simulink model "stp5"  (R2016b)
settings: Solver=VariableStepAuto  StartTime=0.0  StopTime=10.0  RelTol=1e-3
undefined symbols (not defined in the file): Ad2, Bd2, Kd, T, X0
settings Model: Creator=arq  LastModifiedBy=arq

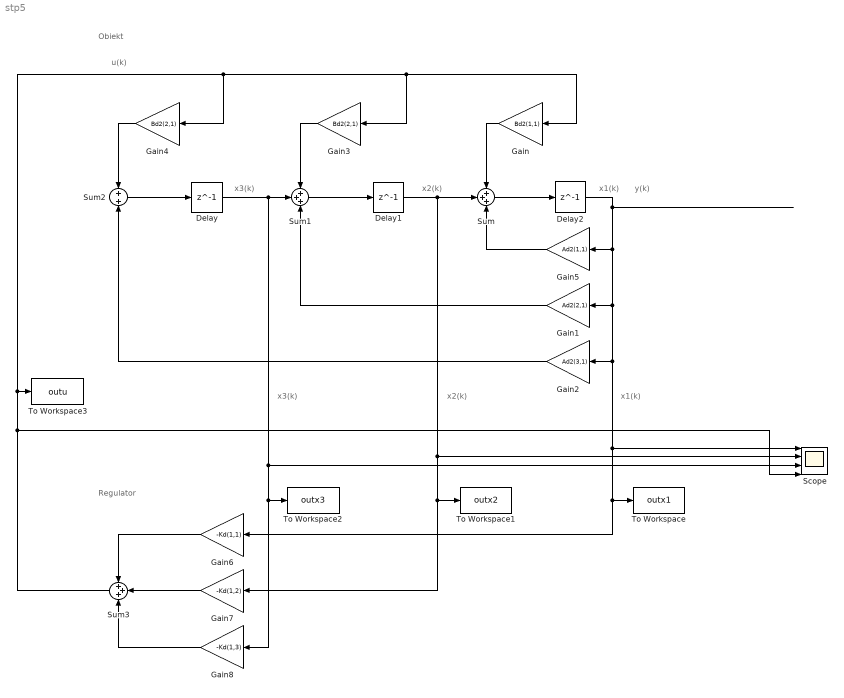
== system stp5 ==
  note: Regulator
  note: Obiekt
  note: u(k)
  note: x3(k)
  note: x2(k)
  note: x1(k)
  note: y(k)
  note: x3(k)
  note: x2(k)
  note: x1(k)
  Delay : Delay  DelayLength=1  InitialCondition=X0(3,1)  SampleTime=T
  Delay1 : Delay  DelayLength=1  InitialCondition=X0(2,1)  SampleTime=T
  Delay2 : Delay  DelayLength=1  InitialCondition=X0(1,1)  SampleTime=T
  Gain : Gain  Gain=Bd2(1,1)
  Gain1 : Gain  Gain=Ad2(2,1)
  Gain2 : Gain  Gain=Ad2(3,1)
  Gain3 : Gain  Gain=Bd2(2,1)
  Gain4 : Gain  Gain=Bd2(2,1)
  Gain5 : Gain  Gain=Ad2(1,1)
  Gain6 : Gain  Gain=-Kd(1,1)
  Gain7 : Gain  Gain=-Kd(1,2)
  Gain8 : Gain  Gain=-Kd(1,3)
  Scope : Scope  NumInputPorts=4
  Sum : Sum  Inputs=3
  Sum1 : Sum  Inputs=3
  Sum2 : Sum  Inputs=2
  Sum3 : Sum  Inputs=+++
  To Workspace : ToWorkspace  VariableName=outx1  SaveFormat=Timeseries  SampleTime=-1
  To Workspace1 : ToWorkspace  VariableName=outx2  SaveFormat=Timeseries  SampleTime=-1
  To Workspace2 : ToWorkspace  VariableName=outx3  SaveFormat=Timeseries  SampleTime=-1
  To Workspace3 : ToWorkspace  VariableName=outu  SaveFormat=Timeseries  SampleTime=-1
  wires:
  Delay2/1 -> Scope/1, Gain6/1, To Workspace/1, Gain2/1, Gain1/1, Gain5/1
  Sum3/1 -> Scope/4, To Workspace3/1, Gain/1, Gain3/1, Gain4/1
  Delay1/1 -> Sum/2, Scope/2, To Workspace1/1, Gain7/1
  Sum/1 -> Delay2/1
  Sum1/1 -> Delay1/1
  Delay/1 -> Scope/3, To Workspace2/1, Gain8/1, Sum1/2
  Gain5/1 -> Sum/3
  Gain1/1 -> Sum1/3
  Gain2/1 -> Sum2/2
  Sum2/1 -> Delay/1
  Gain/1 -> Sum/1
  Gain3/1 -> Sum1/1
  Gain4/1 -> Sum2/1
  Gain6/1 -> Sum3/1
  Gain7/1 -> Sum3/2
  Gain8/1 -> Sum3/3
